simulink model "QuadSearchandRescue"  (R2026a)
settings: Solver=VariableStepDiscrete  MaxStep=Inf
settings Model: DataDictionary=QuadData.sldd  ModifiedByFormat=The MathWorks, Inc.  Creator=The MathWorks, Inc.  LastModifiedBy=The MathWorks, Inc.

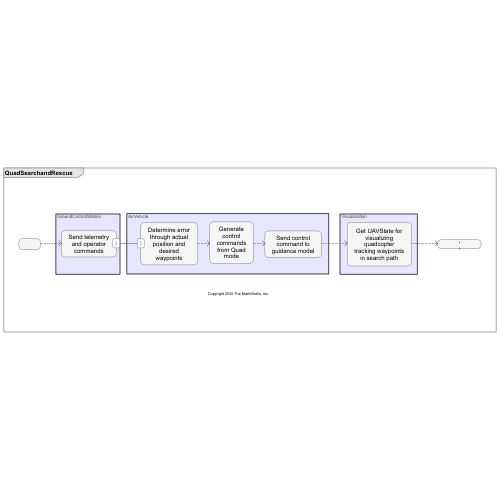
[thumbnail: Simulink's stored preview of the top-level diagram]
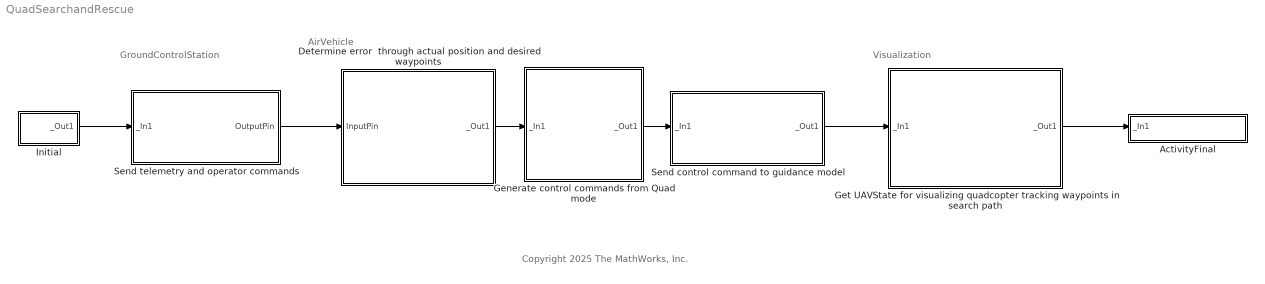
== system QuadSearchandRescue ==
  note: Visualization
  note: AirVehicle
  note: GroundControlStation
  note: Copyright 2025 The MathWorks, Inc.
  ActivityFinal : Subsystem
      settings: CopyFcn=set_param(gcbh,'LinkStatus','none');  PortSchema="{\"entries\":[{\"content\":{\"sides\":[{\"content\":{\"connectorIds\":[\"In1\"]},\"type\":\"ConnectorPlacement.EquallySpacedRectSide\",\"uuid\":\"5b5ee960-3a8a-4ebd-8961-a93e8676becc\"},{\"content\":{\"side\":\"RIGHT\"},\"type\":\"ConnectorPlacement.EquallySpacedRectSide\",\"uuid\":\"056d3e8d-807d-49de-8696-cbe4e7cfdf7b\"},{\"content\":{\"side\":\"TOP\"},\"type\":\"ConnectorPlacement.EquallySpacedRectSide\",\"uuid\":\"90d6e9fa-4419-446a-af19-b3a8e203a514\"}]},\"type\":\"ConnectorPlacement.EquallySpacedConnector\",\"uuid\":\"2cea215f-69c6-419f-8060-567505edb6aa\"}],\"packageUris\":[\"http://schema.mathworks.com/mf0/Connector/R2020b\"],\"version\":\"1.0\"}"
  Determine error  through actual position and desired waypoints : Subsystem
      settings: CopyFcn=set_param(gcbh,'LinkStatus','none');  PortSchema="{\"entries\":[{\"content\":{\"sides\":[{\"content\":{\"connectorIds\":[\"In1\"]},\"type\":\"ConnectorPlacement.EquallySpacedRectSide\",\"uuid\":\"8b8484c1-cf26-4581-b8fc-256a8ecfdb83\"},{\"content\":{\"connectorIds\":[\"Out1\"],\"side\":\"RIGHT\"},\"type\":\"ConnectorPlacement.EquallySpacedRectSide\",\"uuid\":\"3a16a2b5-713c-4388-b877-919135a32b8f\"},{\"content\":{\"side\":\"TOP\"},\"type\":\"ConnectorPlacement.EquallySpacedRectSide\",\"uuid\":\"bed756e8-31b8-4ed2-9d51-3ea7bdc3aaf3\"}]},\"type\":\"ConnectorPlacement.EquallySpacedConnector\",\"uuid\":\"44c99f34-7f08-46c1-84c1-36b9dab88967\"}],\"packageUris\":[\"http://schema.mathworks.com/mf0/Connector/R2020b\"],\"version\":\"1.0\"}"
  Generate control commands from Quad mode : Subsystem
      settings: CopyFcn=set_param(gcbh,'LinkStatus','none');  PortSchema="{\"entries\":[{\"content\":{\"sides\":[{\"content\":{\"connectorIds\":[\"In1\"]},\"type\":\"ConnectorPlacement.EquallySpacedRectSide\",\"uuid\":\"8b8484c1-cf26-4581-b8fc-256a8ecfdb83\"},{\"content\":{\"connectorIds\":[\"Out1\"],\"side\":\"RIGHT\"},\"type\":\"ConnectorPlacement.EquallySpacedRectSide\",\"uuid\":\"3a16a2b5-713c-4388-b877-919135a32b8f\"},{\"content\":{\"side\":\"TOP\"},\"type\":\"ConnectorPlacement.EquallySpacedRectSide\",\"uuid\":\"bed756e8-31b8-4ed2-9d51-3ea7bdc3aaf3\"}]},\"type\":\"ConnectorPlacement.EquallySpacedConnector\",\"uuid\":\"44c99f34-7f08-46c1-84c1-36b9dab88967\"}],\"packageUris\":[\"http://schema.mathworks.com/mf0/Connector/R2020b\"],\"version\":\"1.0\"}"
  Get UAVState for visualizing quadcopter tracking waypoints in search path : Subsystem
      settings: CopyFcn=set_param(gcbh,'LinkStatus','none');  PortSchema="{\"entries\":[{\"content\":{\"sides\":[{\"content\":{\"connectorIds\":[\"In1\"]},\"type\":\"ConnectorPlacement.EquallySpacedRectSide\",\"uuid\":\"8b8484c1-cf26-4581-b8fc-256a8ecfdb83\"},{\"content\":{\"connectorIds\":[\"Out1\"],\"side\":\"RIGHT\"},\"type\":\"ConnectorPlacement.EquallySpacedRectSide\",\"uuid\":\"3a16a2b5-713c-4388-b877-919135a32b8f\"},{\"content\":{\"side\":\"TOP\"},\"type\":\"ConnectorPlacement.EquallySpacedRectSide\",\"uuid\":\"bed756e8-31b8-4ed2-9d51-3ea7bdc3aaf3\"}]},\"type\":\"ConnectorPlacement.EquallySpacedConnector\",\"uuid\":\"44c99f34-7f08-46c1-84c1-36b9dab88967\"}],\"packageUris\":[\"http://schema.mathworks.com/mf0/Connector/R2020b\"],\"version\":\"1.0\"}"
  Initial : Subsystem
      settings: CopyFcn=set_param(gcbh,'LinkStatus','none');  PortSchema="{\"entries\":[{\"content\":{\"sides\":[{\"content\":{},\"type\":\"ConnectorPlacement.EquallySpacedRectSide\",\"uuid\":\"5b5ee960-3a8a-4ebd-8961-a93e8676becc\"},{\"content\":{\"connectorIds\":[\"Out1\"],\"side\":\"RIGHT\"},\"type\":\"ConnectorPlacement.EquallySpacedRectSide\",\"uuid\":\"056d3e8d-807d-49de-8696-cbe4e7cfdf7b\"},{\"content\":{\"side\":\"TOP\"},\"type\":\"ConnectorPlacement.EquallySpacedRectSide\",\"uuid\":\"90d6e9fa-4419-446a-af19-b3a8e203a514\"}]},\"type\":\"ConnectorPlacement.EquallySpacedConnector\",\"uuid\":\"2cea215f-69c6-419f-8060-567505edb6aa\"}],\"packageUris\":[\"http://schema.mathworks.com/mf0/Connector/R2020b\"],\"version\":\"1.0\"}"
  Send control command to guidance model : Subsystem
      settings: CopyFcn=set_param(gcbh,'LinkStatus','none');  PortSchema="{\"entries\":[{\"content\":{\"sides\":[{\"content\":{\"connectorIds\":[\"In1\"]},\"type\":\"ConnectorPlacement.EquallySpacedRectSide\",\"uuid\":\"8b8484c1-cf26-4581-b8fc-256a8ecfdb83\"},{\"content\":{\"connectorIds\":[\"Out1\"],\"side\":\"RIGHT\"},\"type\":\"ConnectorPlacement.EquallySpacedRectSide\",\"uuid\":\"3a16a2b5-713c-4388-b877-919135a32b8f\"},{\"content\":{\"side\":\"TOP\"},\"type\":\"ConnectorPlacement.EquallySpacedRectSide\",\"uuid\":\"bed756e8-31b8-4ed2-9d51-3ea7bdc3aaf3\"}]},\"type\":\"ConnectorPlacement.EquallySpacedConnector\",\"uuid\":\"44c99f34-7f08-46c1-84c1-36b9dab88967\"}],\"packageUris\":[\"http://schema.mathworks.com/mf0/Connector/R2020b\"],\"version\":\"1.0\"}"
  Send telemetry and operator commands : Subsystem
      settings: CopyFcn=set_param(gcbh,'LinkStatus','none');  PortSchema="{\"entries\":[{\"content\":{\"sides\":[{\"content\":{\"connectorIds\":[\"In1\"]},\"type\":\"ConnectorPlacement.EquallySpacedRectSide\",\"uuid\":\"8b8484c1-cf26-4581-b8fc-256a8ecfdb83\"},{\"content\":{\"connectorIds\":[\"Out1\"],\"side\":\"RIGHT\"},\"type\":\"ConnectorPlacement.EquallySpacedRectSide\",\"uuid\":\"3a16a2b5-713c-4388-b877-919135a32b8f\"},{\"content\":{\"side\":\"TOP\"},\"type\":\"ConnectorPlacement.EquallySpacedRectSide\",\"uuid\":\"bed756e8-31b8-4ed2-9d51-3ea7bdc3aaf3\"}]},\"type\":\"ConnectorPlacement.EquallySpacedConnector\",\"uuid\":\"44c99f34-7f08-46c1-84c1-36b9dab88967\"}],\"packageUris\":[\"http://schema.mathworks.com/mf0/Connector/R2020b\"],\"version\":\"1.0\"}"
  wires:
  Initial/1(_Out1) -> Send telemetry and operator commands/1(_In1)
  Generate control commands from Quad mode/1(_Out1) -> Send control command to guidance model/1(_In1)
  Send control command to guidance model/1(_Out1) -> Get UAVState for visualizing quadcopter tracking waypoints in search path/1(_In1)
  Get UAVState for visualizing quadcopter tracking waypoints in search path/1(_Out1) -> ActivityFinal/1(_In1)
  Send telemetry and operator commands/1(OutputPin) -> Determine error  through actual position and desired waypoints/1(InputPin)
  Determine error  through actual position and desired waypoints/1(_Out1) -> Generate control commands from Quad mode/1(_In1)

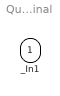
== system QuadSearchandRescue/ActivityFinal ==
  _In1 : Inport

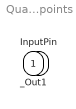
== system QuadSearchandRescue/Determine error  through actual position and desired waypoints ==
  InputPin : Inport
  _Out1 : Outport

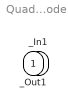
== system QuadSearchandRescue/Generate control commands from Quad mode ==
  _In1 : Inport
  _Out1 : Outport

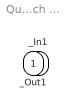
== system QuadSearchandRescue/Get UAVState for visualizing quadcopter tracking waypoints in search path ==
  _In1 : Inport
  _Out1 : Outport

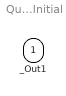
== system QuadSearchandRescue/Initial ==
  _Out1 : Outport

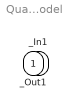
== system QuadSearchandRescue/Send control command to guidance model ==
  _In1 : Inport
  _Out1 : Outport

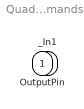
== system QuadSearchandRescue/Send telemetry and operator commands ==
  _In1 : Inport
  OutputPin : Outport  OutDataTypeStr=double  PortDimensions=1
